simulink model "V2X_Core_SRI_coding_rate_symbol"  (R2023b)
settings: Solver=ode23tb  StartTime=0.0  StopTime=50  MaxStep=1e-2  RelTol=1e-3  AbsTol=1e-3
StopFcn:
  | run('saving.m')
values from neighbouring files (symbols this model uses):
  b = 1.6    [a2024_v2x_matlab_6veh.m]
  m = 2000    [a2024_v2x_matlab_6veh.m]
  mEgo = 1500    [a2024_v2x_matlab_6veh.m]
  Mode = 1    [a2024_v2x_matlab_6veh.m]    (also in v2x_matlab.m; v2x_matlabV2.m; v2x_matlab_6veh.m; v2x_matlab_R.m)
  RefSpeed = 90/3.6    (= 25)    [v2x_matlabV2.m]    (also in v2x_matlab_R.m)
  RelDistThreshold = 300    [v2x_matlabV2.m]    (also in v2x_matlab_R.m)
  s = RandStream("dsfmt19937","Seed",15)    [v2x_matlab.m]
  sampleTime = 0.1    [a2024_v2x_matlab_6veh.m]    (also in v2x_matlab.m; v2x_matlabV2.m; v2x_matlab_6veh.m; v2x_matlab_R.m)
  waypoints = [egoWP(:,2) egoWP(:,1), zeroforwp]    [a2024_v2x_matlab_6veh.m]    (also in misc.m = data.data.ActorSpecifications(1,1).Waypoints(:,[1,2]); v2x_matlab.m = data.data.ActorSpecifications(1,1).Waypoints(:,[1,2]); v2x_matlabV2.m = [5 -1.6 0; v2x_matlab_R.m = [5 -1.6 0)
  ZeroActors = struct(     'ActorID',0,     'Position', [1000 1000 1000],      'Velocity', [0 0 0],      'Roll', 0,      'Pitch', 0,      'Yaw', 0,      'AngularVelocity', [0 0 0])    [v2x_matlabV2.m]    (also in v2x_matlab_R.m)
undefined symbols (not defined in the file or in its folder): Battery, Brakes, Control, DiscIntNeverNeededParam, doppler, Drivetrain, ElectricMotor, Env, FB_flag, Init, SNR_value_list, Vehicle, Wheels
libraries: simulink x45, commofdm x29, commdigbbndam3 x15, commchan3 x14, simulink_extras x13, commcnvcod2 x12, commdigbbndpm3 x11, commblkintrlv2 x10, dspmathops x6, sharedtransform x6, autolibutils x6, autolibsharedcoupling x4
(part 6 of 8)

== system V2X_Core_SRI_coding_rate_symbol/VehicleDynamic/DrivetrainControlUnit/Series Regen Braking ==
  note: T / 2 brakes*(muk*pi*Ba^2*Rm*Npads/4)
  note: Changing this to 2 brakes,
      | as HEV motors only braking
      | 1 set of wheels
  note: 1 brakes*(muk*pi*Ba^2*Rm*Npads/4)*P
  note: - Total brake torque request based on brake pressure and parameters of disc brakes
      | - Use as much regenerative motor braking as possible
      | - Any braking torque request that cannot be provided by the motor, will be provided by the friction brakes
  BattSoc : Inport
  VehSpd : Inport  Port=2
  "EMSpd " : Inport  Port=3
  "BrkPrsReq " : Inport  Port=4
  Add : Sum
  ChrgLmt : Lookup_n-D  NumberOfTableDimensions=1  BreakpointsForDimension1=Control.DrivetrainControlUnit.SoCBrakepoints  Table=Control.DrivetrainControlUnit.ChargeLimitBrakepoints  ExtrapMethod=Clip  UseLastTableValue=on  InternalRulePriority=Speed  RndMeth=Simplest
  Constant1 : Constant  Value=2*(Brakes.KineticFrictionCoeff*pi*Brakes.DiskBore^2*Brakes.BrakePadMeanRadius*Brakes.NumPads/4)
  Constant2 : Constant  Value=(Brakes.KineticFrictionCoeff*pi*Brakes.DiskBore^2*Brakes.BrakePadMeanRadius*Brakes.NumPads/4)
  Demux : Demux  Outputs=2
  Demux2 : Demux  Outputs=2
  Gain : Gain  Gain=-1
  Gain6 : Gain  Gain=1/Brakes.MaxPressure
  Gain8 : Gain  Gain=1/Brakes.MaxPressure
  MaxMotTrqVsSpd : Lookup_n-D  NumberOfTableDimensions=1  BreakpointsForDimension1=ElectricMotor.SpeedVector*30/pi  Table=ElectricMotor.TorqueVector  ExtrapMethod=Clip  UseLastTableValue=on  InternalRulePriority=Speed  OutDataTypeStr=Inherit: Inherit from 'Table data'  RndMeth=Simplest
  MinMax : MinMax  Inputs=2
  MotTrqReflectedToWheels : Gain  Gain=Drivetrain.RearDifferential.CarrierToDriveshaftRatio*Drivetrain.EngineToRearDriveshaftRatio
  Negative 5 : Saturate  UpperLimit=inf  LowerLimit=0
  Product{1,3,5..6} (4 alike) : Product
  Product4 : Product  Inputs=*/
  RegenBrakingCutoff : Lookup_n-D  NumberOfTableDimensions=1  BreakpointsForDimension1=Control.DrivetrainControlUnit.RegenBrakingSpeedBrakepoints  Table=Control.DrivetrainControlUnit.RegenBrakingCutoff  ExtrapMethod=Clip  UseLastTableValue=on  InternalRulePriority=Speed  RndMeth=Simplest
  Saturation : Saturate  UpperLimit=1  LowerLimit=0
  Selector : Selector  InputPortWidth=4  IndexOptions=Index vector (dialog)  Indices=[1 2]  OutputSizes=1
  Selector1 : Selector  InputPortWidth=4  IndexOptions=Index vector (dialog)  Indices=[3 4]  OutputSizes=1
  Subtract : Sum  Inputs=+-
  Vector Concatenate : Concatenate  NumInputs=4
  WhlTrqReflectedToMot : Gain  Gain=1/(Drivetrain.RearDifferential.CarrierToDriveshaftRatio*Drivetrain.EngineToRearDriveshaftRatio)
  rads_to_rpm : Gain  Gain=30/pi
  " EMTrqCmdRegen" : Outport  VectorParamsAs1DForOutWhenUnconnected=off
  " BrkCmd" : Outport  Port=2  VectorParamsAs1DForOutWhenUnconnected=off
  wires:
  WhlTrqReflectedToMot/1 -> Gain/1
  Demux/1 -> Vector Concatenate/3
  Gain6/1 -> Saturation/1
  Product1/1 -> Product3/2  "RegenFactor"
  Vector Concatenate/1 -> " BrkCmd"/1
  Demux2/2 -> Product5/2
  Gain8/1 -> Demux/1
  Saturation/1 -> Vector Concatenate/2, Vector Concatenate/1
  ChrgLmt/1 -> Product1/2
  MaxMotTrqVsSpd/1 -> MotTrqReflectedToWheels/1  "MotTrqMax"
  Selector1/1 -> Gain8/1
  Product4/1 -> Gain6/1
  rads_to_rpm/1 -> MaxMotTrqVsSpd/1
  Demux2/1 -> Product6/1
  Product6/1 -> Add/1
  Product5/1 -> Add/2
  Constant1/1 -> Product4/2
  Add/1 -> Subtract/1, MinMax/1  "BrkTrqReqTotal"
  Demux/2 -> Vector Concatenate/4
  "EMSpd "/1 -> rads_to_rpm/1
  RegenBrakingCutoff/1 -> Product1/1
  "BrkPrsReq "/1 -> Selector1/1, Selector/1
  MinMax/1 -> Product3/1  "min"
  Subtract/1 -> Negative 5/1
  MotTrqReflectedToWheels/1 -> MinMax/2  "MotTrqMaxWhls"
  Gain/1 -> " EMTrqCmdRegen"/1  "MotTrqCmdRegen"
  Negative 5/1 -> Product4/1  "BrkTrqFric"
  Selector/1 -> Demux2/1
  BattSoc/1 -> ChrgLmt/1
  VehSpd/1 -> RegenBrakingCutoff/1
  Constant2/1 -> Product6/2, Product5/1
  Product3/1 -> WhlTrqReflectedToMot/1, Subtract/2  "MotTrqRegenWhl"

== system V2X_Core_SRI_coding_rate_symbol/VehicleDynamic/DrivetrainControlUnit/Subsystem2 ==
  SOC : Inport
  Data Type Conversion : DataTypeConversion  SaturateOnIntegerOverflow=off  RndMeth=Floor
  convert2percent : Gain  Gain=100
  BattSOC : Outport
  wires:
  convert2percent/1 -> Data Type Conversion/1
  SOC/1 -> convert2percent/1
  Data Type Conversion/1 -> BattSOC/1

== system V2X_Core_SRI_coding_rate_symbol/VehicleDynamic/FiveSteteABS-TCS/ABSCtrlForEach ==
  Pref : Inport
  WhlAccel : Inport  Port=2
  WhlSlip : Inport  Port=3
  VehSpd : Inport  Port=4
  Constant7 : Constant  Value=WhlAccelOpt
  Constant8 : Constant  Value=KappaOpt
  For Each Subsystem : Subsystem  TreatAsAtomicUnit=on
  Gain : Gain  Gain=Re
  Saturation1 : Saturate  UpperLimit=1  LowerLimit=-1
  Selector : Selector  InputPortWidth=1  IndexOptions=Index vector (dialog)  Indices=[1 1 1 1]  OutputSizes=1
  Sum : Sum  Inputs=|+-
  Sum1 : Sum  Inputs=|+-
  BrkCtrl : Outport
  BrkFlag : Outport  Port=2
  wires:
  Gain/1 -> Sum/1
  Constant8/1 -> Sum1/2
  WhlSlip/1 -> Saturation1/1
  Constant7/1 -> Sum/2
  Sum1/1 -> For Each Subsystem/1(e1)
  WhlAccel/1 -> Gain/1
  Saturation1/1 -> Sum1/1
  For Each Subsystem/2(Flag) -> BrkFlag/1
  Pref/1 -> Selector/1
  VehSpd/1 -> For Each Subsystem/4(VehSpd)
  For Each Subsystem/1(Pb) -> BrkCtrl/1  "BrkPrsCmdCtrl"
  Selector/1 -> For Each Subsystem/3(Pref)
  Sum/1 -> For Each Subsystem/2(e2)

== system V2X_Core_SRI_coding_rate_symbol/VehicleDynamic/FiveSteteABS-TCS/TCSCtrlForEach ==
  WhlAccel : Inport
  WhlSlip : Inport  Port=2
  AccelFdbk : Inport  Port=3
  PbFdbk : Inport  Port=4
  Abs : Abs  SaturateOnIntegerOverflow=off
  Constant7 : Constant  Value=WhlAccelOpt
  Constant8 : Constant  Value=KappaOpt
  Demux : Demux
  For Each Subsystem : Subsystem  TreatAsAtomicUnit=on
  Gain : Gain  Gain=Re
  Gain1 : Gain  Gain=1/2
  Saturation1 : Saturate  UpperLimit=1  LowerLimit=-1
  Selector : Selector  InputPortWidth=1  IndexOptions=Index vector (dialog)  Indices=[1 1 1 1]  OutputSizes=1
  Sum : Sum  Inputs=|+-
  Sum1 : Sum  Inputs=|+-
  Sum2 : Sum  Inputs=++--
  BrkCtrl : Outport
  BrkFlag : Outport  Port=2
  wires:
  Gain/1 -> Sum/1
  Constant8/1 -> Sum1/2
  WhlSlip/1 -> Saturation1/1
  Constant7/1 -> Sum/2
  Sum1/1 -> For Each Subsystem/1(e1)
  WhlAccel/1 -> Gain/1
  Saturation1/1 -> Demux/1, Sum1/1
  For Each Subsystem/2(Flag) -> BrkFlag/1
  AccelFdbk/1 -> Selector/1
  For Each Subsystem/1(Pb) -> BrkCtrl/1  "BrkPrsCmdCtrl"
  Selector/1 -> For Each Subsystem/4(AccelFdbk)
  Sum/1 -> For Each Subsystem/3(e2)
  PbFdbk/1 -> For Each Subsystem/5(PbFdbk)
  Demux/1 -> Sum2/1
  Demux/2 -> Sum2/2
  Demux/3 -> Sum2/3
  Demux/4 -> Sum2/4
  Sum2/1 -> Abs/1
  Abs/1 -> Gain1/1
  Gain1/1 -> For Each Subsystem/2(Enb)

== system V2X_Core_SRI_coding_rate_symbol/VehicleDynamic/FiveSteteABS-TCS/Wheel Accel and Slip Estimator1 ==
  Omega : Inport
  Accel : Inport  Port=2
  Demux : Demux  Outputs=3
  Discrete-Time Integrator : DiscreteIntegrator  IntegratorMethod=Integration: Trapezoidal  SampleTime=-1  ICPrevOutput=DiscIntNeverNeededParam  ICPrevScaledInput=DiscIntNeverNeededParam
  Kappa : Subsystem  TreatAsAtomicUnit=on
  Terminator : Terminator
  Terminator1 : Terminator
  Wheel Accel : Subsystem  TreatAsAtomicUnit=on
  <WhlAccel> : Outport
  <Kappa> : Outport  Port=2
  <xdot> : Outport  Port=3
  wires:
  Accel/1 -> Demux/1
  Discrete-Time Integrator/1 -> <xdot>/1, Kappa/1(xdot)
  Demux/1 -> Discrete-Time Integrator/1
  Demux/2 -> Terminator/1
  Demux/3 -> Terminator1/1
  Omega/1 -> Kappa/2(Omega), Wheel Accel/1(Omega)
  Wheel Accel/1(WhlAccel) -> <WhlAccel>/1
  Kappa/1(KappaEst) -> <Kappa>/1

== system V2X_Core_SRI_coding_rate_symbol/VehicleDynamic/Suspension to Chasiss Transforms/Susp2Body ==
  DCM : Inport
  VehAng : Inport  Port=2
  SuspAng : Inport  Port=3
  Fs : Inport  Port=4  Partition=on  PartitionDimension=2  PartitionWidth=1  PartitionOffset=0
  Ms : Inport  Port=5  Partition=on  PartitionDimension=2  PartitionWidth=1  PartitionOffset=0
  For Each : ForEach  DisableCoverage=on
  Inertial to Body : Product  Multiplication=Matrix(*)  InputSameDT=on  SaturateOnIntegerOverflow=on  OutDataTypeStr=Inherit: Same as first input
  Inertial to Body1 : Product  Multiplication=Matrix(*)  InputSameDT=on  SaturateOnIntegerOverflow=on  OutDataTypeStr=Inherit: Same as first input
  Reshape : Reshape
  Reshape1 : Reshape
  Rotation Angles to Direction Cosine Matrix : sharedtransform/Rotation Angles to Direction Cosine Matrix  rotationOrder=ZYX  aMode=2
  Selector : Selector  InputPortWidth=3  IndexOptions=Index vector (dialog)  Indices=[3 2 1]  OutputSizes=1
  Selector1 : Selector  InputPortWidth=3  IndexOptions=Index vector (dialog)  Indices=[1 2]  OutputSizes=1
  Selector2 : Selector  InputPortWidth=3  IndexOptions=Index vector (dialog)  Indices=[3]  OutputSizes=1
  Transpose : Math  Operator=transpose  SignedPower=on
  Unary Minus : UnaryMinus
  Vector Concatenate : Concatenate
  "transform to Inertial axes " : shared6dof/6DOF (Euler Angles)/transform to Inertial axes   SystemSampleTime=-1  VariantActivationTime=update diagram  AllowFlexibleInterface=on  Latency=0  AutoFrameSizeCalculation=off
  transform to Inertial axes 1 : shared6dof/6DOF (Euler Angles)/transform to Inertial axes   SystemSampleTime=-1  VariantActivationTime=update diagram  AllowFlexibleInterface=on  Latency=0  AutoFrameSizeCalculation=off
  FsB : Outport  ConcatenationDimension=2  VectorParamsAs1DForOutWhenUnconnected=off
  MsB : Outport  Port=2  ConcatenationDimension=2  VectorParamsAs1DForOutWhenUnconnected=off
  wires:
  Reshape/1 -> Inertial to Body/2
  Inertial to Body/1 -> FsB/1
  SuspAng/1 -> Unary Minus/1
  Selector/1 -> Rotation Angles to Direction Cosine Matrix/1
  Fs/1 -> "transform to Inertial axes "/1
  Transpose/1 -> transform to Inertial axes 1/2, "transform to Inertial axes "/2
  Rotation Angles to Direction Cosine Matrix/1 -> Transpose/1
  "transform to Inertial axes "/1 -> Reshape/1
  transform to Inertial axes 1/1 -> Reshape1/1
  Inertial to Body1/1 -> MsB/1
  Reshape1/1 -> Inertial to Body1/2
  DCM/1 -> Inertial to Body1/1, Inertial to Body/1
  Ms/1 -> transform to Inertial axes 1/1
  VehAng/1 -> Selector2/1
  Unary Minus/1 -> Selector1/1
  Selector1/1 -> Vector Concatenate/1
  Vector Concatenate/1 -> Selector/1
  Selector2/1 -> Vector Concatenate/2

== system V2X_Core_SRI_coding_rate_symbol/VehicleDynamic/Tire2Veh/Wheel to Body Transform ==
  Forces : Inport  PortDimensions=[3,1]  Partition=on  PartitionDimension=2  PartitionWidth=1  PartitionOffset=0
  <M> : Inport  Port=2  PortDimensions=[3,1]  Partition=on  PartitionDimension=2  PartitionWidth=1  PartitionOffset=0
  DCM : Inport  Port=3  Partition=on  PartitionDimension=3  PartitionWidth=1  PartitionOffset=0
  <Re> : Inport  Port=4  Partition=on  PartitionDimension=1  PartitionWidth=1  PartitionOffset=0
  WheelAngles : Inport  Port=5  Partition=on  PartitionDimension=2  PartitionWidth=1  PartitionOffset=0
  Add : Sum
  Constant : Constant  Value=[pi;0;0]
  Constant1 : Constant  Value=zeros(2,1)
  Cross Product : matrix_library/Cross Product
  Demux1 : Demux  Outputs=3
  Demux2 : Demux  Outputs=3
  Divide1 : Product  Inputs=***  Multiplication=Matrix(*)
  Divide2 : Product  Inputs=**  Multiplication=Matrix(*)
  Divide3 : Product  Inputs=**  Multiplication=Matrix(*)
  For Each : ForEach  DisableCoverage=on
  Mux : Mux  Inputs=2
  Rotation Angles to Direction Cosine Matrix : sharedtransform/Rotation Angles to Direction Cosine Matrix  rotationOrder=ZYX  aMode=2
  Rotation Angles to Direction Cosine Matrix1 : sharedtransform/Rotation Angles to Direction Cosine Matrix  rotationOrder=ZYX  aMode=2
  Selector : Selector  InputPortWidth=3  IndexOptions=Index vector (dialog)  Indices=[3 2 1]  OutputSizes=1
  Selector1 : Selector  InputPortWidth=3  IndexOptions=Index vector (dialog)  Indices=[3 2 1]  OutputSizes=1
  Transpose : Math  Operator=transpose
  Transpose1 : Math  Operator=transpose
  Fx : Outport  ConcatenationDimension=1  VectorParamsAs1DForOutWhenUnconnected=off
  Fy : Outport  Port=2  ConcatenationDimension=1  VectorParamsAs1DForOutWhenUnconnected=off
  Fz : Outport  Port=3  ConcatenationDimension=1  VectorParamsAs1DForOutWhenUnconnected=off
  Mx : Outport  Port=4  ConcatenationDimension=1  VectorParamsAs1DForOutWhenUnconnected=off
  My : Outport  Port=5  ConcatenationDimension=1  VectorParamsAs1DForOutWhenUnconnected=off
  Mz : Outport  Port=6  ConcatenationDimension=1  VectorParamsAs1DForOutWhenUnconnected=off
  wires:
  Demux1/1 -> Fx/1
  Demux1/2 -> Fy/1
  Demux1/3 -> Fz/1
  Rotation Angles to Direction Cosine Matrix/1 -> Transpose/1
  Forces/1 -> Divide2/2, Cross Product/2
  WheelAngles/1 -> Selector/1
  Selector/1 -> Rotation Angles to Direction Cosine Matrix/1
  Rotation Angles to Direction Cosine Matrix1/1 -> Divide1/3
  Selector1/1 -> Rotation Angles to Direction Cosine Matrix1/1
  Constant/1 -> Selector1/1
  Transpose/1 -> Divide1/2
  DCM/1 -> Transpose1/1
  Transpose1/1 -> Divide1/1
  Divide2/1 -> Demux1/1
  Divide3/1 -> Demux2/1
  Divide1/1 -> Divide3/1, Divide2/1
  <M>/1 -> Add/2
  Demux2/3 -> Mz/1
  Demux2/2 -> My/1
  Demux2/1 -> Mx/1
  Add/1 -> Divide3/2
  Cross Product/1 -> Add/1
  Mux/1 -> Cross Product/1
  <Re>/1 -> Mux/2
  Constant1/1 -> Mux/1

== system V2X_Core_SRI_coding_rate_symbol/VehicleDynamic/Wheel Adapter/Wheel Angles ==
  steer : Inport
  camber : Inport  Port=2
  Constant3 : Constant  Value=ones(1,4).*0
  Reshape : Reshape  OutputDimensionality=Row vector (2-D)
  Reshape1 : Reshape  OutputDimensionality=Row vector (2-D)
  Reshape2 : Reshape  OutputDimensionality=Row vector (2-D)
  Vector Concatenate3 : Concatenate  NumInputs=3  Mode=Multidimensional array
  Vehicle : Outport  VectorParamsAs1DForOutWhenUnconnected=off
  wires:
  Constant3/1 -> Reshape2/1
  Vector Concatenate3/1 -> Vehicle/1
  Reshape/1 -> Vector Concatenate3/3
  Reshape1/1 -> Vector Concatenate3/1
  camber/1 -> Reshape1/1
  Reshape2/1 -> Vector Concatenate3/2
  steer/1 -> Reshape/1

== system V2X_Core_SRI_coding_rate_symbol/VehicleDynamic/Wheel Adapter/Wheel to Body Transform ==
  VelVeh : Inport  Partition=on  PartitionDimension=2  PartitionWidth=1  PartitionOffset=0
  WheelAngles : Inport  Port=2  Partition=on  PartitionDimension=2  PartitionWidth=1  PartitionOffset=0
  Constant : Constant  Value=[pi;0;0]
  Demux1 : Demux  Outputs=3
  Divide1 : Product  Inputs=**  Multiplication=Matrix(*)
  Divide2 : Product  Inputs=**  Multiplication=Matrix(*)
  For Each : ForEach  DisableCoverage=on
  Rotation Angles to Direction Cosine Matrix : sharedtransform/Rotation Angles to Direction Cosine Matrix  rotationOrder=ZYX  aMode=2
  Rotation Angles to Direction Cosine Matrix1 : sharedtransform/Rotation Angles to Direction Cosine Matrix  rotationOrder=ZYX  aMode=2
  Selector : Selector  InputPortWidth=3  IndexOptions=Index vector (dialog)  Indices=[3 2 1]  OutputSizes=1
  Selector1 : Selector  InputPortWidth=3  IndexOptions=Index vector (dialog)  Indices=[3 2 1]  OutputSizes=1
  xdotWheel : Outport  ConcatenationDimension=1  VectorParamsAs1DForOutWhenUnconnected=off
  ydotWheel : Outport  Port=2  ConcatenationDimension=1  VectorParamsAs1DForOutWhenUnconnected=off
  zdotWheel : Outport  Port=3  ConcatenationDimension=1  VectorParamsAs1DForOutWhenUnconnected=off
  wires:
  Divide2/1 -> Demux1/1
  Demux1/1 -> xdotWheel/1
  Demux1/2 -> ydotWheel/1
  Demux1/3 -> zdotWheel/1
  Rotation Angles to Direction Cosine Matrix/1 -> Divide1/1
  VelVeh/1 -> Divide1/2
  WheelAngles/1 -> Selector/1
  Selector/1 -> Rotation Angles to Direction Cosine Matrix/1
  Selector1/1 -> Rotation Angles to Direction Cosine Matrix1/1
  Rotation Angles to Direction Cosine Matrix1/1 -> Divide2/1
  Divide1/1 -> Divide2/2
  Constant/1 -> Selector1/1

== system V2X_Core_SRI_coding_rate_symbol/VehicleDynamic/Wheel Adapter/scale factors with friction ==
  lamda_mu_x : Inport
  lamda_mu_y : Inport  Port=2
  0 : Constant  Value=[zeros(1,numWheels)]  VectorParams1D=off
  1 : Constant  Value=[zeros(2,numWheels)]+1  VectorParams1D=off
  2 : Constant  Value=[zeros(1,numWheels)]+1  VectorParams1D=off
  Reshape : Reshape  OutputDimensionality=Row vector (2-D)  OutputDimensions=[1,numWheels]
  Reshape1 : Reshape  OutputDimensionality=Row vector (2-D)  OutputDimensions=[1,numWheels]
  Signal Specification3 : SignalSpecification  Unit=1
  Vector Concatenate : Concatenate  NumInputs=9  Mode=Multidimensional array
  ones : Constant  Value=[ones(6,numWheels)]  VectorParams1D=off
  ones1 : Constant  Value=[ones(9,numWheels)]  VectorParams1D=off
  ones2 : Constant  Value=ones(1,numWheels)  VectorParams1D=off
  ones3 : Constant  Value=[ones(5,numWheels)]  VectorParams1D=off
  lambdas : Outport  Unit=1  VectorParamsAs1DForOutWhenUnconnected=off
  wires:
  lamda_mu_y/1 -> Reshape1/1
  lamda_mu_x/1 -> Reshape/1
  ones2/1 -> Vector Concatenate/1  "lambda_Fz0"
  Vector Concatenate/1 -> Signal Specification3/1
  ones/1 -> Vector Concatenate/9
  0/1 -> Vector Concatenate/4  "lamda_mu_V"
  Reshape1/1 -> Vector Concatenate/3
  Reshape/1 -> Vector Concatenate/2
  Signal Specification3/1 -> lambdas/1
  1/1 -> Vector Concatenate/8  "lam_Vykappa"
  ones1/1 -> Vector Concatenate/5
  2/1 -> Vector Concatenate/6  "lam_Vy"
  ones3/1 -> Vector Concatenate/7

== system V2X_Core_SRI_coding_rate_symbol/VehicleDynamic/AccelerationToTrq/CalculateIntendedTorque/Acceleration Resistance Torque ==
  note: AccTrq=Mass*acc*rStat
  IntendedLongAcc[m/s**2] : Inport
  EngInrt[kg*m**2] : Inport  Port=2
  WheelRotAxisInrt[kg*m**2] : Inport  Port=3
  OverallMass[kg] : Inport  Port=4
  UnloadedTireRadius[m] : Inport  Port=5
  TorqueRatio[-] : Inport  Port=6
  Divide1 : Product  Inputs=*/
  Divide2 : Product  Inputs=**
  Divide3 : Product  Inputs=*/
  Gain : Gain  Gain=0.25
  Mass[kg] : Sum  Inputs=+++
  Product1 : Product  Inputs=3  RndMeth=Zero
  Product2 : Product  Inputs=3  RndMeth=Zero
  Sum of Elements : Sum  Inputs=+
  Sum of Elements1 : Sum  Inputs=+
  AccResistanceTrq[Nm] : Outport  VectorParamsAs1DForOutWhenUnconnected=off
  wires:
  Sum of Elements1/1 -> Mass[kg]/1
  Divide1/1 -> Product2/2, Product2/1
  Product1/1 -> AccResistanceTrq[Nm]/1
  Gain/1 -> Divide1/2, Product1/3
  OverallMass[kg]/1 -> Mass[kg]/3
  UnloadedTireRadius[m]/1 -> Divide2/1, Divide2/2, Sum of Elements/1
  TorqueRatio[-]/1 -> Divide1/1
  Sum of Elements/1 -> Gain/1
  Mass[kg]/1 -> Product1/1
  Product2/1 -> Mass[kg]/2
  IntendedLongAcc[m/s**2]/1 -> Product1/2
  Divide3/1 -> Sum of Elements1/1
  WheelRotAxisInrt[kg*m**2]/1 -> Divide3/1
  Divide2/1 -> Divide3/2
  EngInrt[kg*m**2]/1 -> Product2/3

== system V2X_Core_SRI_coding_rate_symbol/VehicleDynamic/AccelerationToTrq/CalculateIntendedTorque/Driving Resistance Torque ==
  note: Reibverluste dazu addieren
  note: all resistances must be positive!
  note: Mresistance=Mincline+Mdrag+Mroll
  UnloadedTireRadius[m] : Inport
  TireMaxRollResistanceTrq[Nm] : Inport  Port=2
  AeroFrc(VehSys)[N] : Inport  Port=3
  Add : Sum  Inputs=++++
  FrictionLoss[Nm] : Constant  Value=0
  Gain : Gain  Gain=-1
  Gain1 : Gain  Gain=-1
  Gain2 : Gain  Gain=0.25
  Mincline [Nm] : Constant  Value=0
  Product : Product  RndMeth=Zero
  Sum of Elements : Sum  Inputs=+
  Sum of Elements1 : Sum  Inputs=+
  DrivingResistanceTrq[Nm] : Outport  VectorParamsAs1DForOutWhenUnconnected=off
  wires:
  FrictionLoss[Nm]/1 -> Add/4
  Gain2/1 -> Product/2
  Sum of Elements1/1 -> Gain1/1
  Sum of Elements/1 -> Gain2/1
  Mincline [Nm]/1 -> Add/1
  UnloadedTireRadius[m]/1 -> Sum of Elements/1
  Gain/1 -> Product/1
  Add/1 -> DrivingResistanceTrq[Nm]/1
  TireMaxRollResistanceTrq[Nm]/1 -> Sum of Elements1/1
  Product/1 -> Add/3
  AeroFrc(VehSys)[N]/1 -> Gain/1
  Gain1/1 -> Add/2

== system V2X_Core_SRI_coding_rate_symbol/VehicleDynamic/AccelerationToTrq/CalculateIntendedTorque/Reference Torque ==
  note: Intercept "division-by-zero" when
      | ideling and no gear is chosen
  note: Mengine,req=(Maccel+Mres)/iGes
  AccResistanceTrq[Nm] : Inport
  TorqueRatio[-] : Inport  Port=2
  DrivingResistanceTrq[Nm] : Inport  Port=3
  MinEngTrq[Nm] : Inport  Port=4
  Add : Sum
  Divide : Product  Inputs=*/
  NonZero : DriverAssistanceSystemsModules/AdaptiveCruiseControlUnit/ACCController/CalculateIntendedTorque/Reference Torque/NonZero  Commented=on  NonZero=0.001
  NonZero1 : Subsystem
  Switch2 : Switch  Criteria=u2 ~= 0  SaturateOnIntegerOverflow=off  InputSameDT=off
  checkForAlmostZero : Subsystem
  IntendedTrq[Nm] : Outport  VectorParamsAs1DForOutWhenUnconnected=off
  wires:
  AccResistanceTrq[Nm]/1 -> Add/1
  checkForAlmostZero/1(Out1) -> Switch2/2
  TorqueRatio[-]/1 -> NonZero1/1(Input), checkForAlmostZero/1(In1)
  DrivingResistanceTrq[Nm]/1 -> Add/2
  Divide/1 -> Switch2/3
  Switch2/1 -> IntendedTrq[Nm]/1
  MinEngTrq[Nm]/1 -> Switch2/1  "Ratio=0: RefTrq"
  Add/1 -> Divide/1
  NonZero1/1(Output) -> Divide/2

== system V2X_Core_SRI_coding_rate_symbol/VehicleDynamic/AccelerationToTrq/CalculateMainBrakePressure/NonZero ==
  Input : Inport
  Constant : Constant  Value=0
  Constant1 : Constant  Value=0.001
  Relational Operator : RelationalOperator  Operator=~=
  Switch : Switch  Threshold=0.5
  Output : Outport  VectorParamsAs1DForOutWhenUnconnected=off
  wires:
  Input/1 -> Switch/1, Relational Operator/1
  Relational Operator/1 -> Switch/2
  Constant1/1 -> Switch/3
  Constant/1 -> Relational Operator/2
  Switch/1 -> Output/1

== system V2X_Core_SRI_coding_rate_symbol/VehicleDynamic/DrivetrainControlUnit/Motor Torque Arbitration and Power Management/Power Management ==
  note: Power Management algorithm:
      | - Estimate Elec power based on mech power using efficiency map
      | - Check if Elec power is within battery power limits
      | - If power within limit , use motor torque command
      | - If power limit exceeded, use limited motor torque
      | - For low Mot Spd, MotPwrReq will be a small number.  Pass through torque command until Mot Spd > 2.
  BattPwrDischrgLmt : Inport
  BattPwrChrgLmt : Inport  Port=2
  EMSpd : Inport  Port=3
  EMTrqCmd : Inport  Port=4
  SOC : Inport  Port=5
  Abs : Abs  SaturateOnIntegerOverflow=off
  Check Within Limits : Subsystem
  Compare To Constant : simulink/Logic and Bit Operations/Compare To Constant  relop=<  const=2  OutDataTypeStr=boolean
  ElecToMechPwr : Product  Inputs=*/
  Mech to Elec Power Estimate : Subsystem
  MechPwrToTrq : Product  Inputs=*/
  Switch : Switch  Criteria=u2 > Threshold  SaturateOnIntegerOverflow=off  InputSameDT=off
  Switch1 : Switch  Criteria=u2 > Threshold  SaturateOnIntegerOverflow=off  InputSameDT=off
  Torque Limit : Subsystem
  div0protect - poly : autolibutils/div0protect - poly  thresh=2  ZeroCross1=off  aMode=6
  EMTrqCmdFinal : Outport  VectorParamsAs1DForOutWhenUnconnected=off
  wires:
  EMSpd/1 -> Abs/1, Torque Limit/2(EMSpd), div0protect - poly/1, Mech to Elec Power Estimate/2(EMSpd)
  EMTrqCmd/1 -> Switch/1, Switch1/1, Mech to Elec Power Estimate/1(EMTrqCmd)
  div0protect - poly/1 -> MechPwrToTrq/2
  Mech to Elec Power Estimate/2(Eff2k) -> ElecToMechPwr/2
  ElecToMechPwr/1 -> MechPwrToTrq/1
  MechPwrToTrq/1 -> Switch/3
  Torque Limit/1(EMTrqCmd) -> EMTrqCmdFinal/1
  BattPwrDischrgLmt/1 -> Check Within Limits/1(up)
  Mech to Elec Power Estimate/1(EMPwrElecReq) -> Check Within Limits/2(u)
  BattPwrChrgLmt/1 -> Check Within Limits/3(lo)
  Check Within Limits/2(y) -> ElecToMechPwr/1
  Switch/1 -> Switch1/3
  Check Within Limits/1(InLimit) -> Switch/2
  Switch1/1 -> Torque Limit/1(EMTrq)
  Abs/1 -> Compare To Constant/1
  Compare To Constant/1 -> Switch1/2
  SOC/1 -> Torque Limit/3(SOC)

== system V2X_Core_SRI_coding_rate_symbol/VehicleDynamic/FiveSteteABS-TCS/ABSCtrlForEach/For Each Subsystem ==
  e1 : Inport  Partition=on  PartitionDimension=1  PartitionWidth=1  PartitionOffset=0
  e2 : Inport  Port=2  Partition=on  PartitionDimension=1  PartitionWidth=1  PartitionOffset=0
  Pref : Inport  Port=3  Partition=on  PartitionDimension=1  PartitionWidth=1  PartitionOffset=0
  VehSpd : Inport  Port=4
  ABSForEachWheel : Stateflow chart  InitFcn=[~]=vehdynicon('vehdynblk',gcb);  TreatAsAtomicUnit=on
  For Each : ForEach  DisableCoverage=on
  Saturation2 : Saturate  UpperLimit=1  LowerLimit=0  ZeroCross=off
  Pb : Outport  ConcatenationDimension=1
  Flag : Outport  Port=2  ConcatenationDimension=1
  wires:
  e1/1 -> ABSForEachWheel/1(e1)
  e2/1 -> ABSForEachWheel/2(e2)
  VehSpd/1 -> ABSForEachWheel/4(VehSpd)
  Saturation2/1 -> Pb/1  "BrkPrsCmdCtrl"
  ABSForEachWheel/2(Flag) -> Flag/1
  ABSForEachWheel/1(PbOutput) -> Saturation2/1
  Pref/1 -> ABSForEachWheel/3(Pref)

== system V2X_Core_SRI_coding_rate_symbol/VehicleDynamic/FiveSteteABS-TCS/TCSCtrlForEach/For Each Subsystem ==
  e1 : Inport  Partition=on  PartitionDimension=1  PartitionWidth=1  PartitionOffset=0
  Enb : Inport  Port=2
  e2 : Inport  Port=3  Partition=on  PartitionDimension=1  PartitionWidth=1  PartitionOffset=0
  AccelFdbk : Inport  Port=4  Partition=on  PartitionDimension=1  PartitionWidth=1  PartitionOffset=0
  PbFdbk : Inport  Port=5  Partition=on  PartitionDimension=1  PartitionWidth=1  PartitionOffset=0
  ABSForEachWheel : Stateflow chart  InitFcn=[~]=vehdynicon('vehdynblk',gcb);  TreatAsAtomicUnit=on
  Discrete-Time Integrator1 : DiscreteIntegrator  IntegratorMethod=Integration: Trapezoidal  ExternalReset=rising  SampleTime=-1  LimitOutput=on  UpperSaturationLimit=1  LowerSaturationLimit=0  ICPrevOutput=DiscIntNeverNeededParam  ICPrevScaledInput=DiscIntNeverNeededParam
  For Each : ForEach  DisableCoverage=on
  IsNegative : simulink/Logic and Bit Operations/Compare To Zero  relop===  OutDataTypeStr=boolean  ZeroCross=off
  Pb : Outport  ConcatenationDimension=1
  Flag : Outport  Port=2  ConcatenationDimension=1
  wires:
  e1/1 -> ABSForEachWheel/1(e1)
  e2/1 -> ABSForEachWheel/2(e2)
  Discrete-Time Integrator1/1 -> Pb/1  "BrkPrsCmdCtrl"
  ABSForEachWheel/2(Flag) -> IsNegative/1, Flag/1
  ABSForEachWheel/1(PbOutput) -> Discrete-Time Integrator1/1
  AccelFdbk/1 -> ABSForEachWheel/3(AccelFdbk)
  Enb/1 -> ABSForEachWheel/4(Enb)
  PbFdbk/1 -> ABSForEachWheel/5(Pb)
  IsNegative/1 -> Discrete-Time Integrator1/2

== system V2X_Core_SRI_coding_rate_symbol/VehicleDynamic/FiveSteteABS-TCS/Wheel Accel and Slip Estimator1/Kappa ==
  xdot : Inport
  Omega : Inport  Port=2  PortDimensions=1  Partition=on  PartitionDimension=1  PartitionWidth=1  PartitionOffset=0
  For Each : ForEach  DisableCoverage=on
  MATLAB Function : MATLAB Function  TreatAsAtomicUnit=on
  KappaEst : Outport  ConcatenationDimension=1
  wires:
  MATLAB Function/1(KappaEst) -> KappaEst/1
  xdot/1 -> MATLAB Function/2(xdot)
  Omega/1 -> MATLAB Function/1(Omega)

== system V2X_Core_SRI_coding_rate_symbol/VehicleDynamic/FiveSteteABS-TCS/Wheel Accel and Slip Estimator1/Wheel Accel ==
  Omega : Inport  PortDimensions=1  Partition=on  PartitionDimension=1  PartitionWidth=1  PartitionOffset=0
  For Each : ForEach  DisableCoverage=on
  SG Diff : autolibutils/SG Diff  N=2  F=500  div0Tol=.001  aMode=2
  Terminator : Terminator
  WhlAccel : Outport  ConcatenationDimension=1
  wires:
  Omega/1 -> SG Diff/1
  SG Diff/1 -> Terminator/1
  SG Diff/2 -> WhlAccel/1

== system V2X_Core_SRI_coding_rate_symbol/VehicleDynamic/AccelerationToTrq/CalculateIntendedTorque/Reference Torque/NonZero1 ==
  Input : Inport
  Constant : Constant  Value=0
  Constant1 : Constant  Value=0.001
  Relational Operator : RelationalOperator  Operator=~=
  Switch : Switch  Threshold=0.5
  Output : Outport  VectorParamsAs1DForOutWhenUnconnected=off
  wires:
  Input/1 -> Switch/1, Relational Operator/1
  Relational Operator/1 -> Switch/2
  Constant1/1 -> Switch/3
  Constant/1 -> Relational Operator/2
  Switch/1 -> Output/1

== system V2X_Core_SRI_coding_rate_symbol/VehicleDynamic/AccelerationToTrq/CalculateIntendedTorque/Reference Torque/checkForAlmostZero ==
  note: Todo!
  In1 : Inport
  Compare To Constant1 : simulink/Logic and Bit Operations/Compare To Constant  relop=<=  const=1e-6  OutDataTypeStr=boolean  ZeroCross=off
  Out1 : Outport  VectorParamsAs1DForOutWhenUnconnected=off
  wires:
  In1/1 -> Compare To Constant1/1
  Compare To Constant1/1 -> Out1/1

== system V2X_Core_SRI_coding_rate_symbol/VehicleDynamic/DrivetrainControlUnit/Motor Torque Arbitration and Power Management/Power Management/Check Within Limits ==
  up : Inport
  u : Inport  Port=2
  lo : Inport  Port=3
  Compare To Zero : simulink/Logic and Bit Operations/Compare To Zero  relop=>=  OutDataTypeStr=boolean
  Compare To Zero1 : simulink/Logic and Bit Operations/Compare To Zero  relop=<=  OutDataTypeStr=boolean
  Logical Operator : Logic  AllPortsSameDT=off  OutDataTypeStr=boolean
  Saturation Dynamic1 : simulink/Discontinuities/Saturation Dynamic  OutMin=[]  OutMax=[]  OutDataTypeStr=Inherit: Same as second input  OutDataType=fixdt(1, 16)  OutScaling=2^-10  DoSatur=off
  Subtract : Sum  Inputs=+-
  Subtract1 : Sum  Inputs=-+
  InLimit : Outport  VectorParamsAs1DForOutWhenUnconnected=off
  y : Outport  Port=2  VectorParamsAs1DForOutWhenUnconnected=off
  wires:
  Saturation Dynamic1/1 -> y/1
  lo/1 -> Subtract1/2, Saturation Dynamic1/3
  up/1 -> Subtract/1, Saturation Dynamic1/1
  u/1 -> Subtract1/1, Subtract/2, Saturation Dynamic1/2
  Subtract/1 -> Compare To Zero/1
  Subtract1/1 -> Compare To Zero1/1
  Compare To Zero/1 -> Logical Operator/1
  Compare To Zero1/1 -> Logical Operator/2
  Logical Operator/1 -> InLimit/1

== system V2X_Core_SRI_coding_rate_symbol/VehicleDynamic/DrivetrainControlUnit/Motor Torque Arbitration and Power Management/Power Management/Mech to Elec Power Estimate ==
  note: Check if Motoring
      | or Generating
  note: Using an Efficiency Map, we can estimate the
      | Electric Power from the Mechanical  Torque Request.
  note: Pelec_req = Pmech_req*Eff^k,
      | k = -1 if Motoring >= 0,
      | k = 1 if Generating < 0
  EMTrqCmd : Inport
  EMSpd : Inport  Port=2
  Abs : Abs  SaturateOnIntegerOverflow=off
  Abs1 : Abs  SaturateOnIntegerOverflow=off
  Constant1 : Constant  Value=-1  SampleTime=-1
  Constant2 : Constant  SampleTime=-1
  Eff Map : Lookup_n-D  BreakpointsForDimension1=ElectricMotor.SpeedVector*30/pi  BreakpointsForDimension2=ElectricMotor.TorqueEfficiencyVector  Table=ElectricMotor.EfficiencyTable  ExtrapMethod=Clip  UseLastTableValue=on  InternalRulePriority=Speed  OutDataTypeStr=Inherit: Inherit from 'Table data'  RndMeth=Simplest
      settings: InputPortMap=u0,u1
  Gain1 : Gain  Gain=1/100
  Math Function : Math  Operator=pow  SignedPower=on  OutputSignalType=real
  Product : Product
  Product3 : Product
  Product4 : Product
  Switch2 : Switch  SaturateOnIntegerOverflow=off  InputSameDT=off
  rads_to_rpm : Gain  Gain=30/pi
  EMPwrElecReq : Outport  VectorParamsAs1DForOutWhenUnconnected=off
  Eff2k : Outport  Port=2  VectorParamsAs1DForOutWhenUnconnected=off
  wires:
  Product3/1 -> Product4/1
  Switch2/1 -> Math Function/2
  Constant1/1 -> Switch2/1
  Constant2/1 -> Switch2/3
  Eff Map/1 -> Gain1/1
  Abs/1 -> Eff Map/1
  Gain1/1 -> Math Function/1
  Math Function/1 -> Eff2k/1, Product4/2
  Product4/1 -> EMPwrElecReq/1
  Abs1/1 -> Eff Map/2
  rads_to_rpm/1 -> Abs/1
  Product/1 -> Switch2/2
  EMSpd/1 -> Product3/1, Product/1, rads_to_rpm/1
  EMTrqCmd/1 -> Product3/2, Product/2, Abs1/1

== system V2X_Core_SRI_coding_rate_symbol/VehicleDynamic/DrivetrainControlUnit/Motor Torque Arbitration and Power Management/Power Management/Torque Limit ==
  EMTrq : Inport
  EMSpd : Inport  Port=2
  SOC : Inport  Port=3
  Compare To Constant : simulink/Logic and Bit Operations/Compare To Constant  relop=>  const=1  OutDataTypeStr=boolean
  Constant : Constant  Value=0
  Gain : Gain  Gain=-1
  MaxEMTrqVsSpd : Lookup_n-D  NumberOfTableDimensions=1  BreakpointsForDimension1=ElectricMotor.SpeedVector  Table=ElectricMotor.TorqueVector  ExtrapMethod=Clip  UseLastTableValue=on  InternalRulePriority=Speed  OutDataTypeStr=Inherit: Inherit from 'Table data'  RndMeth=Simplest
  Saturation Dynamic : simulink/Discontinuities/Saturation Dynamic  OutMin=[]  OutMax=[]  OutDataTypeStr=Inherit: Same as second input  OutDataType=fixdt(1, 16)  OutScaling=2^-10  DoSatur=off
  Switch : Switch  Criteria=u2 > Threshold  SaturateOnIntegerOverflow=off  InputSameDT=off
  rads_to_rpm : Gain  Gain=30/pi
  EMTrqCmd : Outport  VectorParamsAs1DForOutWhenUnconnected=off
  wires:
  EMTrq/1 -> Saturation Dynamic/2
  Saturation Dynamic/1 -> EMTrqCmd/1
  EMSpd/1 -> rads_to_rpm/1
  MaxEMTrqVsSpd/1 -> Gain/1, Switch/1
  rads_to_rpm/1 -> MaxEMTrqVsSpd/1
  Gain/1 -> Saturation Dynamic/3
  SOC/1 -> Compare To Constant/1
  Compare To Constant/1 -> Switch/2
  Constant/1 -> Switch/3
  Switch/1 -> Saturation Dynamic/1

== matlab function V2X_Core_SRI_coding_rate_symbol/DSRC/Subsystem3/MATLAB Function2 ==
  settings: sampleTime=sampleTime
  data: input input; Actors output
function Actors = getRealValues(input) 

modulated = input;

NumActors = modulated(1,:);
Time = modulated(2,:);

ActorID = modulated(3,1);

posMultip = 10;  % 10
posX = (modulated(4,:)/posMultip);
posY = (modulated(5,:)/posMultip);
posZ = (modulated(6,:)/posMultip);

velMultip = 50;  % 50
vX = (modulated(7,:)/velMultip);
vY = (modulated(8,:)/velMultip);
vZ = (modulated(9,:)/velMultip);

rpyMultip = 50;  % 50
Roll = (modulated(10,:)/rpyMultip);
Pitch = (modulated(11,:)/rpyMultip);
Yaw = (modulated(12,:)/rpyMultip);

angvelMultip = 50;  % 50
angularVelocityX = (modulated(13,:)/angvelMultip);
angularVelocityY = (modulated(14,:)/angvelMultip);
angularVelocityZ = (modulated(15,:)/angvelMultip);

% Velocity = [vX vY vZ];
% Position = [posX posY posZ];
% AngularVelocity = [angularVelocityX; angularVelocityY; angularVelocityZ];


%Actors = [NumActors; Time; ActorID; Position; Velocity; Roll; Pitch; Yaw; AngularVelocity];
Actors = double([NumActors; Time; ActorID; posX; posY; posZ; vX; vY; vZ; Roll; Pitch; Yaw; angularVelocityX; angularVelocityY; angularVelocityZ]);


end

== matlab function V2X_Core_SRI_coding_rate_symbol/VehicleDynamic/MATLAB Function2 ==
  data: RefSpeed input; RefSpeedMax output; v_HV input; v_RV input; pdr input; lat input; sri_target input
function RefSpeedMax = calculate_SRI_max_speed(RefSpeed, v_HV, v_RV, pdr, lat, sri_target)

%V_HV_UPPER_LIMIT = 1.0
%V_HV_LOWER_LIMIT = 0.0
SRI_TARGET = 0.1;
DEFAULT_HV_SPEED = 190 / 3.6; % in m/s
DEFAULT_RV_SPEED =  190 / 3.6; % in m/s

OLSparams = [0.1283, -0.0089, -0.2621, -0.0181, 0.6640, -0.0156, -0.2030, -1.1130, 0.3615, 0.1294, 0.5597, 0.1044, 0.0613, -0.5524, 0.0934];



    pdr_norm = pdr / 100;
    lat_norm = lat / 1000;
    v_HV_norm = v_HV / DEFAULT_HV_SPEED;
    v_RV_norm = v_RV / DEFAULT_RV_SPEED;
    sri_val =   OLSparams(1) ...
            + OLSparams(2)  * v_HV_norm ...
            + OLSparams(3)  * v_RV_norm ...
            + OLSparams(4)  * pdr_norm ...
            + OLSparams(5)  * v_HV_norm^2 ...
            + OLSparams(6)  * v_RV_norm^2 ...
            + OLSparams(7)  * v_RV_norm * pdr_norm ...
            + OLSparams(8)  * pdr_norm * (v_HV_norm^2) ...
            + OLSparams(9)  * pdr_norm * (v_RV_norm^2) ...
            + OLSparams(10) * lat_norm * (v_HV_norm^2) ...
            + OLSparams(11) * (v_HV_norm^2) * (pdr_norm^2) ...
            + OLSparams(12) * v_HV_norm * v_RV_norm * lat_norm ...
            + OLSparams(13) * v_RV_norm * pdr_norm * lat_norm ...
            + OLSparams(14) * v_RV_norm * lat_norm * (v_HV_norm^2)...
            + OLSparams(15) * lat_norm * (v_HV_norm^2) * (v_RV_norm^2);
    % sri_val = SRI_value(v_HV_normalized,v_RV_normalized, pdr_normalized, lat_normalized);
    if sri_val <= sri_target
        RefSpeedMax = RefSpeed;
    else
        lb0 = 0.0;
        ub0 = v_HV_norm;
        x0 = 1.0;
        %value_bounds = Bounds([V_HV_LOWER_LIMIT],[v_HV_normalized])

        sri_err_fun = @(v_HV_norm) abs(OLSparams(1) ...
                                    + OLSparams(2)  * v_HV_norm ...
                                    + OLSparams(3)  * v_RV_norm ...
                                    + OLSparams(4)  * pdr_norm ...
                                    + OLSparams(5)  * v_HV_norm^2 ...
                                    + OLSparams(6)  * v_RV_norm^2 ...
                                    + OLSparams(7)  * v_RV_norm * pdr_norm ...
                                    + OLSparams(8)  * pdr_norm * (v_HV_norm^2) ...
                                    + OLSparams(9)  * pdr_norm * (v_RV_norm^2) ...
                                    + OLSparams(10) * lat_norm * (v_HV_norm^2) ...
                                    + OLSparams(11) * (v_HV_norm^2) * (pdr_norm^2) ...
                                    + OLSparams(12) * v_HV_norm * v_RV_norm * lat_norm ...
                                    + OLSparams(13) * v_RV_norm * pdr_norm * lat_norm ...
                                    + OLSparams(14) * v_RV_norm * lat_norm * (v_HV_norm^2)...
                                    + OLSparams(15) * lat_norm * (v_HV_norm^2) * (v_RV_norm^2) ...
                                    - SRI_TARGET);
        % sri_err_fun = @(v_HV_norm) abs(SRI_value(v_HV_norm, v_RV_normalized, pdr_normalized, lat_normalized) - SRI_TARGET);
        opts = optimoptions('fmincon','Algorithm','sqp');
        [v_HV_max_normalized] = fmincon(sri_err_fun, x0,[], [],[],[], lb0, ub0, [], opts);
        %res = minimize(fun=SRI_target_function, x0=[1.0], bounds=value_bounds, args=(v_RV_normalized, pdr_normalized, lat_normalized, sri_target))
        %v_HV_max_normalized = res.x[0];
        RefSpeedMax = v_HV_max_normalized*DEFAULT_HV_SPEED; % in m/s
    end

end


% 
% 
% % 
% % v_HV_0 = 0.0;
% % SRI_target = 0.5;
% % v_RV = v_RV_original / (50.0/3.6);
% % 
% % OLSparams = [0.1283, -0.0089, -0.2621, -0.0181, 0.6640, -0.0156, -0.2030, -1.1130, 0.3615, 0.1294, 0.5597, 0.1044, 0.0613, -0.5524, 0.0934];
% % 
% % 
% % SRI = @(v_HV) abs(OLSparams(1) ...
% %                 + OLSparams(2) * PDR ...
% %                 + OLSparams(3) * LAT ...
% %                 + OLSparams(4) * v_HV ...
% %                 + OLSparams(5) * v_HV^2 ...
% %                 + OLSparams(6) * PDR * v_HV ...
% %                 + OLSparams(7) * PDR * v_RV ...
% %                 + OLSparams(8) * v_HV * v_RV^2 ...
% %                 + OLSparams(9) * v_RV * v_HV^2 ...
% %                 + OLSparams(10) * PDR * v_RV * v_HV^2 ...
% %                 + OLSparams(11) * PDR^2 * v_HV * v_RV^2 ...
% %                 + OLSparams(12) * PDR^2 * v_HV^2 * v_RV ...
% %                 + OLSparams(13) * PDR^2 * v_HV^2*v_RV^2 ...
% %                 - SRI_target);
% %  v_HV = fminsearch(SRI, v_HV_0) * 130.0/3.6;
% % end
% % 
% % 
% % from scipy.optimize import minimize, Bounds
% % from time import perf_counter
% %

== matlab function V2X_Core_SRI_coding_rate_symbol/Vehicle 3/MATLAB Function2 ==
  data: busActors3Test1 input; intVector output int16 size=15; VehicleID input
  events: trigger input RISING_EDGE_EVENT
function intVector = convBus2IntVector(busActors3Test1, VehicleID)

% Data extracted from actorss bus

%ActorId = BusActors1Actors.Actors(ActorID).ActorID(1:1);
numActors = busActors3Test1.NumActors;
time = busActors3Test1.Time;

ActorID = VehicleID;

posX = busActors3Test1.Actors(ActorID).Position(1:1);
posY = busActors3Test1.Actors(ActorID).Position(2:2);
posZ = busActors3Test1.Actors(ActorID).Position(3:3);

vX = busActors3Test1.Actors(ActorID).Velocity(1:1);
vY = busActors3Test1.Actors(ActorID).Velocity(2:2);
vZ = busActors3Test1.Actors(ActorID).Velocity(3:3);

roll = busActors3Test1.Actors(ActorID).Roll(1:1);
pitch = busActors3Test1.Actors(ActorID).Pitch(1:1);
yaw = busActors3Test1.Actors(ActorID).Yaw(1:1);


angularVelocityX = busActors3Test1.Actors(ActorID).AngularVelocity(1:1);
angularVelocityY = busActors3Test1.Actors(ActorID).AngularVelocity(2:2);
angularVelocityZ = busActors3Test1.Actors(ActorID).AngularVelocity(3:3);


% Converting the data

ActorID = int16(ActorID);

posMultip = 10;
posX = int16(round(posMultip*posX));
posY = int16(round(posMultip*posY));
posZ = int16(round(posMultip*posZ));

velMultip = 50;
vX = int16(round(velMultip * vX));
vY = int16(round(velMultip * vY));
vZ = int16(round(velMultip * vZ));

rpyMultip = 50;
roll = int16(round(rpyMultip * roll));
pitch = int16(round(rpyMultip * pitch));
yaw = int16(round(rpyMultip * yaw));

angvelMultip = 50;
angularVelocityX = int16(round(angvelMultip * angularVelocityX));
angularVelocityY = int16(round(angvelMultip * angularVelocityY));
angularVelocityZ = int16(round(angvelMultip * angularVelocityZ));


% Output vector
%zerosVector = zeros(9,1);

intVector = [numActors; time; ActorID; posX; posY; posZ; vX; vY; vZ; roll; pitch; yaw; angularVelocityX; angularVelocityY; angularVelocityZ];
end

== matlab function V2X_Core_SRI_coding_rate_symbol/Subsystem1/MATLAB Function1 ==
  data: busActors3Test1 input; Actor output int16 size=15; VehicleID input; VehicleData output Bus: Actors; EgoData input Bus: Actors; counter output
  events: trigger input RISING_EDGE_EVENT
function [Actor, VehicleData, counter]  = convBus2IntVector(busActors3Test1, VehicleID, EgoData)

% Data extracted from actorss bus

%ActorId = BusActors1Actors.Actors(ActorID).ActorID(1:1);
numActors = busActors3Test1.NumActors;
%time = busActors3Test1.Time;
time = busActors3Test1.Time;

ActorID = VehicleID;

posX = busActors3Test1.Actors(ActorID).Position(1:1);
posY = busActors3Test1.Actors(ActorID).Position(2:2);
posZ = busActors3Test1.Actors(ActorID).Position(3:3);
vPos = [posX posY posZ];

vX = busActors3Test1.Actors(ActorID).Velocity(1:1);
vY = busActors3Test1.Actors(ActorID).Velocity(2:2);
vZ = busActors3Test1.Actors(ActorID).Velocity(3:3);

roll = busActors3Test1.Actors(ActorID).Roll(1:1);
pitch = busActors3Test1.Actors(ActorID).Pitch(1:1);
yaw = busActors3Test1.Actors(ActorID).Yaw(1:1);


angularVelocityX = busActors3Test1.Actors(ActorID).AngularVelocity(1:1);
angularVelocityY = busActors3Test1.Actors(ActorID).AngularVelocity(2:2);
angularVelocityZ = busActors3Test1.Actors(ActorID).AngularVelocity(3:3);

VehicleData = busActors3Test1.Actors(ActorID);


%% Converting the data

ActorID = int16(ActorID);

posMultip = 10;
posX = int16(round(posMultip*posX));
posY = int16(round(posMultip*posY));
posZ = int16(round(posMultip*posZ));

velMultip = 50;
vX = int16(round(velMultip * vX));
vY = int16(round(velMultip * vY));
vZ = int16(round(velMultip * vZ));

rpyMultip = 50;
roll = int16(round(rpyMultip * roll));
pitch = int16(round(rpyMultip * pitch));
yaw = int16(round(rpyMultip * yaw));

angvelMultip = 50;
angularVelocityX = int16(round(angvelMultip * angularVelocityX));
angularVelocityY = int16(round(angvelMultip * angularVelocityY));
angularVelocityZ = int16(round(angvelMultip * angularVelocityZ));


% Output vector
%zerosVector = zeros(9,1);

intVector = [numActors; time; ActorID; posX; posY; posZ; vX; vY; vZ; roll; pitch; yaw; angularVelocityX; angularVelocityY; angularVelocityZ];



%% Pathloss (freespace)

EgoPos = EgoData.Position;
dist = norm(vPos - EgoPos);

fc = 5.9*10^9;  % Carrier frequency
lambda = physconst('LightSpeed')/fc;

PL = fspl(dist, lambda);

Pt_dBm = 33;    % [dBm] Transmission power; maximum permissible transmit power level
sigma = rand(1) + 3.2;  % [3.7 +- 0.5] Variance of the shadowing effect in the wireless communication channel
                        % shadowing follows a log-normal random distribution
X = randn(1);       % random variable following a normal distribution with mean 0 and standard deviation 1
SH = sigma * X;

Pr = Pt_dBm - PL - SH;

P_SEN = -60;

ZeroActors = int16(zeros(15,1));

persistent prev_value;
if isempty(prev_value)
    prev_value = ZeroActors; % Initialize to a default value
end

if Pr > P_SEN
    Actor = intVector;
    prev_value = intVector;
else
    Actor = prev_value;
end


%% Packet counter
counter = 0;

if (Pr > P_SEN)
    counter = counter + 1;
end


end

== matlab function V2X_Core_SRI_coding_rate_symbol/Perception/Choosing target  ==
  settings: updateMethod=DISCRETE  sampleTime=0.1
  data: ActorsMX input; RelDist output double size=1; RelVel output; EgoData input
function [RelDist, RelVel] = extractLeadInfo(ActorsMX, EgoData)

ActorID = 1; % Ego vehicle ID
% RelDist = 101;
% RelVel = 101;

%% 1. Actors and Egos positon, yaw, and velocity from the incoming data

threshold_dist = 100; % meter
numColumns = size(ActorsMX, 2);  % = the number of vehicles in the scenario - the ego vehicle

ActorsMXpos = double(ActorsMX(4:6,:));   % extracting only the positions
ActorsMXyaw = double(ActorsMX(12,:));   % extracting only the yaw
%ActorsMxvel = double(ActorsMX(7:9,2:end));

% Extracting the position, velocity and yaw of the ego


EgoPos = (double(EgoData.Position))';
EgoVel = double(EgoData.Velocity)';

EgoPosNorm = norm(double(EgoData.Position));
EgoVelNorm = norm(double(EgoData.Velocity));
 
if EgoVelNorm == 0
    EgoVelNorm = 16;
end
EgoYaw = double(deg2rad(EgoData.Yaw));


%% 2. Create a new matrix to store the filtered columns
filteredActorsMX = NaN(size(ActorsMX));
filteredColumnCount = 0;  % Initialize the count of filtered columns


%% 3. Filter the columns to keep the actor only
egoActoriDist = zeros(1,numColumns); % initialize the distance between ego and lead vehicle
egoActoriYaw = zeros(1,numColumns);  % initialize the yaw differnece between ego and lead vehicle

% disp(EgoPosNorm)
% disp(norm(ActorsMXpos(:, 3)))

for i = 1:numColumns
    egoActoriDist(:,i) = norm(ActorsMXpos(:, i)) - EgoPosNorm;
end
%disp(egoActoriDist)
for i = 1:numColumns
    egoActoriYaw(:,i) = ActorsMXyaw(:,i) - EgoYaw;
end

for i = 1:numColumns
     if ActorsMX(3,i) == 1
        %  (abs(egoActoriDist(:,i)) <= threshold_dist) && ...
        % (abs(egoActoriYaw(:,i)) <= 20)
            
        % If the column meets the criteria, copy it to the new matrix
        filteredColumnCount = filteredColumnCount + 1;
        filteredActorsMX(:, filteredColumnCount) = ActorsMX(:,i);
    end
end

% Remove any columns filled with NaN values in filteredActorsMX
filteredActorsMX = filteredActorsMX(:, ~all(isnan(filteredActorsMX)));
filteredActorsMX(:, ~any(filteredActorsMX)) = [];

persistent prev_vel prev_dist;
if isempty(prev_vel)
    prev_vel = 10; % Initialize to a default value
end
if isempty(prev_dist)
    prev_dist = 100; % Initialize to a default value
end



if ~isempty(filteredActorsMX) 
    LeadPos = filteredActorsMX(4:6,1);
    %LeadPosNorm = norm(LeadPos);
    LeadVel = filteredActorsMX(7:9,1);
    LeadVelNorm = norm(LeadVel);
    %disp(filteredActorsMX(1,:));
    RelDist1 =  norm(LeadPos - EgoPos);
    RelVel1 =  LeadVelNorm - EgoVelNorm;
    if ((-500 <= RelDist1) && (RelDist1 <= 500) && (-200 <= RelVel1) && (RelVel1 <= 200))
        RelDist = RelDist1;
        RelVel = RelVel1;
        prev_vel = RelVel1;
        prev_dist = RelDist1;
    else
        RelDist = prev_dist;
        RelVel = prev_vel;
    end
else
    % Handle the case when filteredActorsMX is empty
    RelDist = prev_dist;
    RelVel = prev_vel;
end



end

== matlab function V2X_Core_SRI_coding_rate_symbol/DSRC/Subsystem/MATLAB Function2 ==
  settings: updateMethod=DISCRETE  sampleTime=sampleTime
  data: modulated input; signal output; SNR input
function signal = PRO_error(modulated, SNR)

signal = awgn(modulated,SNR, -7);
